simulink model "Delay_Model"  (R2023a)
settings: Solver=VariableStepAuto  StartTime=0.0  StopTime=10.0  RelTol=1e-3
libraries: NSA_DEVS_LOGISTICS_ATOMIC x2, NSA_DEVS_SINKS_ATOMIC x2, NSA_DEVS_SOURCES_ATOMIC x1
settings Model: Creator=david  LastModifiedBy=david

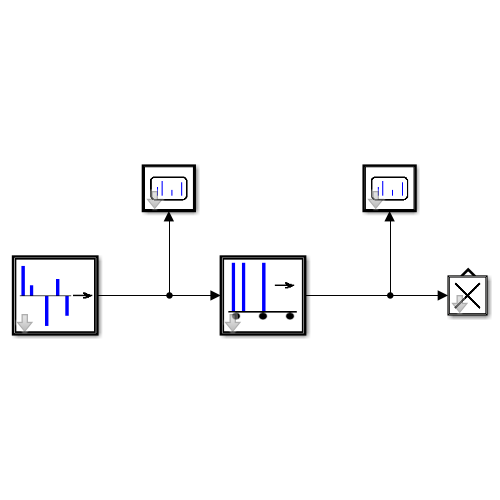
[thumbnail: Simulink's stored preview of the top-level diagram]
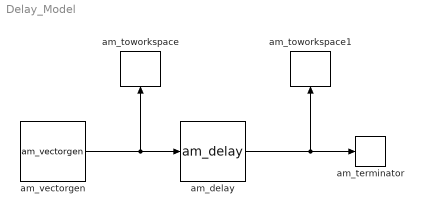
== system Delay_Model ==
  am_delay : NSA_DEVS_LOGISTICS_ATOMIC/am_delay  dt=2  tau=[0,1]  debug=0
      settings: SourceProductName=NSA_DEVS
  am_terminator : NSA_DEVS_LOGISTICS_ATOMIC/am_terminator  tau=[0,1]  debug=0
      settings: SourceProductName=NSA_DEVS
  am_toworkspace : NSA_DEVS_SINKS_ATOMIC/am_toworkspace  varname="\"genOut\""  t0=0  format="\"vector\""  tau=[0,5]  debug=0
      settings: SourceProductName=NSA_DEVS
  am_toworkspace1 : NSA_DEVS_SINKS_ATOMIC/am_toworkspace  varname="\"DelayOut\""  t0=0  format="\"vector\""  tau=[0,5]  debug=0
      settings: SourceProductName=NSA_DEVS
  am_vectorgen : NSA_DEVS_SOURCES_ATOMIC/am_vectorgen  tvec=[1, 3, 7, 8, 9]  yvec=[2, -3, 2, -2, -1]  tau=[0,1]  debug=0
      settings: SourceProductName=NSA_DEVS
  wires:
  am_vectorgen/1 -> am_toworkspace/1, am_delay/1
  am_delay/1 -> am_toworkspace1/1, am_terminator/1
